simulink model "Questao_2"  (R2023b)
settings: Solver=VariableStepAuto  StartTime=0.0  StopTime=50  RelTol=1e-3
settings Model: Creator=pedro  LastModifiedBy=pedro

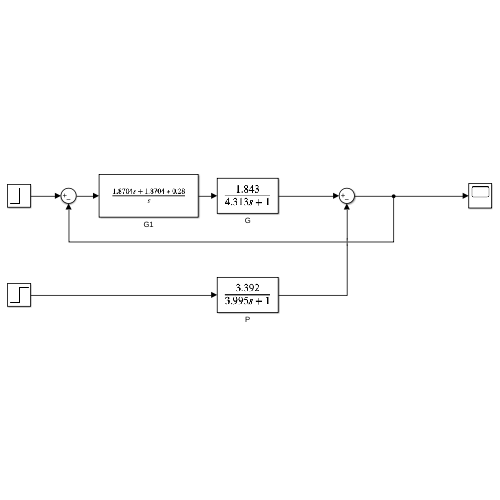
[thumbnail: Simulink's stored preview of the top-level diagram]
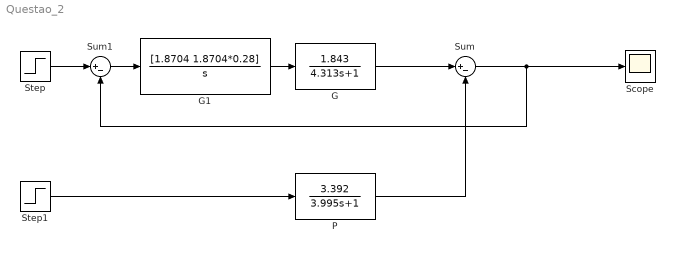
== system Questao_2 ==
  G : TransferFcn  Numerator=[1.843]  Denominator=[4.313 1]
  G1 : TransferFcn  Numerator=[1.8704 1.8704*0.28]  Denominator=[1 0]
  P : TransferFcn  Numerator=[3.392]  Denominator=[3.995 1]
  Scope : Scope
  Step : Step  SampleTime=0
  Step1 : Step  Time=10  SampleTime=0
  Sum : Sum  Inputs=|+-
  Sum1 : Sum  Inputs=|+-
  wires:
  P/1 -> Sum/2
  G/1 -> Sum/1
  Sum/1 -> Sum1/2, Scope/1
  Step1/1 -> P/1
  Step/1 -> Sum1/1
  G1/1 -> G/1
  Sum1/1 -> G1/1
